simulink subsystem "clarkinv"  (R2020a)
settings: Solver=VariableStepAuto  StartTime=0.0  StopTime=10.0  RelTol=1e-3
settings Model: Creator=ZhuanZ（无密码）  LastModifiedBy=ZhuanZ（无密码）

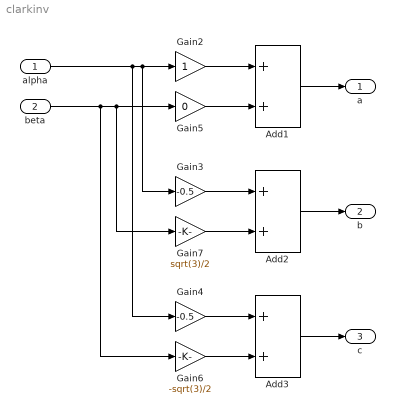
== system clarkinv ==
  alpha : Inport
  beta : Inport  Port=2
  Add1 : Sum
  Add2 : Sum
  Add3 : Sum
  Gain2 : Gain
  Gain3 : Gain  Gain=-0.5
  Gain4 : Gain  Gain=-0.5
  Gain5 : Gain  Gain=0
  Gain6 : Gain  Gain=-sqrt(3)/2
  Gain7 : Gain  Gain=sqrt(3)/2
  a : Outport
  b : Outport  Port=2
  c : Outport  Port=3
  wires:
  Gain2/1 -> Add1/1
  Gain5/1 -> Add1/2
  Gain3/1 -> Add2/1
  Gain7/1 -> Add2/2
  Gain4/1 -> Add3/1
  Gain6/1 -> Add3/2
  beta/1 -> Gain6/1, Gain7/1, Gain5/1
  alpha/1 -> Gain4/1, Gain3/1, Gain2/1
  Add1/1 -> a/1
  Add2/1 -> b/1
  Add3/1 -> c/1
